simulink model "IEEE_39bus_genout"  (R2021a)
settings: Solver=ode3  StartTime=0.0  StopTime=100  FixedStep=Ts  MaxStep=1/60  RelTol=1e-2  AbsTol=1e-1
PreLoadFcn:
  | Ts=50e-6; ssn_ieee39_params; dec=20;
InitFcn:
  | Ts=50e-6; ssn_ieee39_params; dec=20;
values from neighbouring files (symbols this model uses):
  f = 50    [ssn_ieee39_params_ctrl.m]
  fNom = f    (= 60)    [ssn_ieee39_params_ctrl.m]
  ILR = 5.02    [ssn_ieee39_params_ctrl.m]
  IQMIN = 0.1    [ssn_ieee39_params_ctrl.m]
  ISCLIM = 1    [ssn_ieee39_params_ctrl.m]
  ITFpu = 1.10    (= 1.1)    [ssn_ieee39_params_ctrl.m]
  K = 1    [ssn_ieee39_params_ctrl.m]
  K1 = 1    [ssn_ieee39_params_ctrl.m]
  K2 = 2    [ssn_ieee39_params_ctrl.m]
  KCL = 1.04    [ssn_ieee39_params_ctrl.m]
  KFB = 0    [ssn_ieee39_params_ctrl.m]
  KFF = 1    [ssn_ieee39_params_ctrl.m]
  KFIX = 1    [ssn_ieee39_params_ctrl.m]
  KG = 1    [ssn_ieee39_params_ctrl.m]
  KIA = 59.91    [ssn_ieee39_params_ctrl.m]
  KIOEX = 0.0303    [ssn_ieee39_params_ctrl.m]
  KIUEX = 0.0303    [ssn_ieee39_params_ctrl.m]
  KIUOEX = 1    [ssn_ieee39_params_ctrl.m]
  KIUUEX = 1    [ssn_ieee39_params_ctrl.m]
  KLR = 22.47    [ssn_ieee39_params_ctrl.m]
  KM = 1    [ssn_ieee39_params_ctrl.m]
  KOEL = 0.24    [ssn_ieee39_params_ctrl.m]
  Kp = 1    [ssn_ieee39_params_ctrl.m]
  KPA = 30    [ssn_ieee39_params_ctrl.m]
  KPOEL = 1    [ssn_ieee39_params_ctrl.m]
  KPOEX = 0    [ssn_ieee39_params_ctrl.m]
  KPUEX = 0    [ssn_ieee39_params_ctrl.m]
  KSCALE = 0.319    [ssn_ieee39_params_ctrl.m]
  KUF = 0    [ssn_ieee39_params_ctrl.m]
  KUI = 0.001    [ssn_ieee39_params_ctrl.m]
  KUL = 0.24    [ssn_ieee39_params_ctrl.m]
  s = 10    [ssn_ieee39_params_ctrl.m]
  TA = 0.01    [ssn_ieee39_params_ctrl.m]
  Tadj = 0    [ssn_ieee39_params_ctrl.m]
  taps = [1 1 1.07 1.07 1.009 1.025 1 1.025 1.025 1.025]*1    [ssn_ieee39_params_ctrl.m]
  TF = 0.02    [ssn_ieee39_params_ctrl.m]
  TG = 0.024    [ssn_ieee39_params_ctrl.m]
  TINV = 0    [ssn_ieee39_params_ctrl.m]
  TIT = 0.1    [ssn_ieee39_params_ctrl.m]
  TL_10_11_len = 14    [ssn_ieee39_params_ctrl.m]
  TL_10_13_len = 14    [ssn_ieee39_params_ctrl.m]
  TL_13_14_len = 32    [ssn_ieee39_params_ctrl.m]
  TL_14_15_len = 70    [ssn_ieee39_params_ctrl.m]
  TL_15_16_len = 31.5    [ssn_ieee39_params_ctrl.m]
  TL_16_17_len = 26    [ssn_ieee39_params_ctrl.m]
  TL_16_19_len = 61    [ssn_ieee39_params_ctrl.m]
  TL_16_21_len = 46    [ssn_ieee39_params_ctrl.m]
  TL_16_24_len = 15    [ssn_ieee39_params_ctrl.m]
  TL_17_18_len = 26    [ssn_ieee39_params_ctrl.m]
  TL_17_27_len = 59    [ssn_ieee39_params_ctrl.m]
  TL_1_2_len = 134    [ssn_ieee39_params_ctrl.m]
  TL_1_39_len = 105    [ssn_ieee39_params_ctrl.m]
  TL_21_22_len = 47    [ssn_ieee39_params_ctrl.m]
  TL_22_23_len = 33    [ssn_ieee39_params_ctrl.m]
  TL_24_23_len = 88    [ssn_ieee39_params_ctrl.m]
  TL_25_26_len = 101    [ssn_ieee39_params_ctrl.m]
  TL_26_27_len = 46.5    [ssn_ieee39_params_ctrl.m]
  TL_26_28_len = 151    [ssn_ieee39_params_ctrl.m]
  TL_26_29_len = 200    [ssn_ieee39_params_ctrl.m]
  TL_28_29_len = 48    [ssn_ieee39_params_ctrl.m]
  TL_2_25_len = 28    [ssn_ieee39_params_ctrl.m]
  TL_2_2_len = 49    [ssn_ieee39_params_ctrl.m]
  TL_3_18_len = 42    [ssn_ieee39_params_ctrl.m]
  TL_3_4_len = 53    [ssn_ieee39_params_ctrl.m]
  TL_4_14_len = 33    [ssn_ieee39_params_ctrl.m]
  TL_4_5_len = 32.5    [ssn_ieee39_params_ctrl.m]
  TL_5_6_len = 14    [ssn_ieee39_params_ctrl.m]
  TL_5_8_len = 32    [ssn_ieee39_params_ctrl.m]
  TL_6_11_len = 26.5    [ssn_ieee39_params_ctrl.m]
  TL_6_7_len = 25.5    [ssn_ieee39_params_ctrl.m]
  TL_7_8_len = 15    [ssn_ieee39_params_ctrl.m]
  TL_8_9_len = 93    [ssn_ieee39_params_ctrl.m]
  TL_9_39_len = 136    [ssn_ieee39_params_ctrl.m]
  TOEL = 5.00    (= 5)    [ssn_ieee39_params_ctrl.m]
  TQREF = 0    [ssn_ieee39_params_ctrl.m]
  TQSCL = 0.012    [ssn_ieee39_params_ctrl.m]
  Ts_PMU = 1/1000    (= 0.001)    [ssn_ieee39_params_ctrl.m]
  TU1 = 0    [ssn_ieee39_params_ctrl.m]
  TU2 = 0    [ssn_ieee39_params_ctrl.m]
  TU3 = 0    [ssn_ieee39_params_ctrl.m]
  TU4 = 0    [ssn_ieee39_params_ctrl.m]
  TUL = 0    [ssn_ieee39_params_ctrl.m]
  TUP = 0.050    (= 0.05)    [ssn_ieee39_params_ctrl.m]
  TUQ = .005    (= 0.005)    [ssn_ieee39_params_ctrl.m]
  TUV = 0.2    [ssn_ieee39_params_ctrl.m]
  VAAMAX = VAMAX    (= 7.05)    [ssn_ieee39_params_ctrl.m]
  VAMAX = 7.05    [ssn_ieee39_params_ctrl.m]
  VAMIN = -6.11    [ssn_ieee39_params_ctrl.m]
  VBMAX = 999    [ssn_ieee39_params_ctrl.m]
  VF = 0    [ssn_ieee39_params_ctrl.m]
  VFB = 0    [ssn_ieee39_params_ctrl.m]
  VMMAX = 7.05    [ssn_ieee39_params_ctrl.m]
  VMMIN = -6.11    [ssn_ieee39_params_ctrl.m]
  VOELmax1 = 0.2353    [ssn_ieee39_params_ctrl.m]
  VOELmax2 = 0.0    (= 0)    [ssn_ieee39_params_ctrl.m]
  VOELmin1 = -0.24    [ssn_ieee39_params_ctrl.m]
  VOELmin2 = -1.0    (= -1)    [ssn_ieee39_params_ctrl.m]
  VRMAX = 7.05    [ssn_ieee39_params_ctrl.m]
  VRMIN = -6.11    [ssn_ieee39_params_ctrl.m]
  VSCLmax = 0.20    (= 0.2)    [ssn_ieee39_params_ctrl.m]
  VSCLmin = -0.10    (= -0.1)    [ssn_ieee39_params_ctrl.m]
  VUELmax1 = 1    [ssn_ieee39_params_ctrl.m]
  VUELmax2 = 1    [ssn_ieee39_params_ctrl.m]
  VUELmin1 = -1    [ssn_ieee39_params_ctrl.m]
  VUELmin2 = -1    [ssn_ieee39_params_ctrl.m]
  VUImax = 1    [ssn_ieee39_params_ctrl.m]
  VUImin = -1    [ssn_ieee39_params_ctrl.m]
undefined symbols (not defined in the file or in its folder): D1, Delta, MOV_segment9, powergui
libraries: spsThreePhaseVIMeasurementLib x42, slpidlib x40, powerlib_extras x30, op_dpl_lib x30, simulink_extras x20, spsST2AModel x20, spsThreePhaseParallelRLCLoadLib x19, spsThreePhaseTransformerTwoWindingsLib x13, spsSynchronousMachinepuStandardLib x10, simulink x10, spsPower3phInstantaneousLib x10, spsThreePhasePISectionLineLib x7
(part 6 of 12)

== system IEEE_39bus_genout/powergui/EquivalentModel4/Yout ==
  v,i : Inport
  Demux : Demux  Outputs=[2 1 1 1 1 1 1 1 1 1 1 1 1 1 1 1 1 1 1]
  tag scope: T61_5349_5543534420475=global, T61_5350_5545816817448=global, T61_5351_5548253508191=global, T61_5378_5534547660656=global, T61_5379_5536455134372=global, T61_5380_5538914352885=global, T62_5427_5653550607702=global, T62_5428_5655608975241=global, T62_5429_5658223434786=global, T73_6528_8854035683177=global, T83_7198_10636597834129=global, T83_7199_10636984207108=global, T83_7200_10631654038889=global, T83_7200_10637604369245=global, T83_7201_10632036892151=global, T83_7202_10632653534569=global, T84_7253_10872805404045=global, T84_7254_10873268569375=global, T84_7255_10873968878514=global
  wires:
  v,i/1 -> Demux/1
  Demux/1 -> [T73_6528_8854035683177]
  Demux/2 -> [T61_5378_5534547660656]
  Demux/3 -> [T61_5380_5538914352885]
  Demux/4 -> [T61_5379_5536455134372]
  Demux/5 -> [T62_5427_5653550607702]
  Demux/6 -> [T62_5429_5658223434786]
  Demux/7 -> [T62_5428_5655608975241]
  Demux/8 -> [T83_7198_10636597834129]
  Demux/9 -> [T83_7199_10636984207108]
  Demux/10 -> [T83_7200_10637604369245]
  Demux/11 -> [T84_7253_10872805404045]
  Demux/12 -> [T84_7254_10873268569375]
  Demux/13 -> [T84_7255_10873968878514]
  Demux/14 -> [T83_7200_10631654038889]
  Demux/15 -> [T83_7201_10632036892151]
  Demux/16 -> [T83_7202_10632653534569]
  Demux/17 -> [T61_5349_5543534420475]
  Demux/18 -> [T61_5350_5545816817448]
  Demux/19 -> [T61_5351_5548253508191]

== system IEEE_39bus_genout/powergui/EquivalentModel5/Sources ==
  Mux : Mux  Inputs=[1 1 1 1 1 1 1 1 1]
  u : Outport  VectorParamsAs1DForOutWhenUnconnected=off
  wires:
  Mux/1 -> u/1
  [T82_6942_9370736474068] -> Mux/1
  [T82_6943_9371870963565] -> Mux/2
  [T82_6944_9373248380867] -> Mux/3
  [T82_6945_9366351637990] -> Mux/4
  [T82_6946_9367479825753] -> Mux/5
  [T82_6947_9368850941320] -> Mux/6
  [T81_6895_9154721531022] -> Mux/7
  [T81_6896_9155759447410] -> Mux/8
  [T81_6897_9157036925528] -> Mux/9

== system IEEE_39bus_genout/powergui/EquivalentModel5/Yout ==
  v,i : Inport
  Demux : Demux  Outputs=[1 1 1 1 1 1 1 1 1 1 1 1]
  tag scope: T62_5429_5650937724339=global, T62_5430_5652992041777=global, T62_5431_5655602216520=global, T84_7253_10872378862689=global, T84_7254_10872842362976=global, T84_7255_10873543007073=global, T85_7300_11128438027275=global, T85_7301_11128992896359=global, T85_7302_11129788264501=global, T85_7303_11122740902331=global, T85_7304_11123289832852=global, T85_7305_11124079262431=global
  wires:
  v,i/1 -> Demux/1
  Demux/1 -> [T62_5429_5650937724339]
  Demux/2 -> [T62_5431_5655602216520]
  Demux/3 -> [T62_5430_5652992041777]
  Demux/4 -> [T85_7300_11128438027275]
  Demux/5 -> [T85_7301_11128992896359]
  Demux/6 -> [T85_7302_11129788264501]
  Demux/7 -> [T85_7303_11122740902331]
  Demux/8 -> [T85_7304_11123289832852]
  Demux/9 -> [T85_7305_11124079262431]
  Demux/10 -> [T84_7253_10872378862689]
  Demux/11 -> [T84_7254_10872842362976]
  Demux/12 -> [T84_7255_10873543007073]

== system IEEE_39bus_genout/powergui/EquivalentModel6/Sources ==
  Mux : Mux  Inputs=[1 1 1 1 1 1]
  u : Outport  VectorParamsAs1DForOutWhenUnconnected=off
  wires:
  Mux/1 -> u/1
  [T80_6854_8930207033252] -> Mux/1
  [T80_6855_8931137197264] -> Mux/2
  [T80_6856_8932303557277] -> Mux/3
  [T81_6907_9133741612475] -> Mux/4
  [T81_6908_9134756992429] -> Mux/5
  [T81_6909_9136011934111] -> Mux/6

== system IEEE_39bus_genout/powergui/EquivalentModel6/Yout ==
  v,i : Inport
  Demux : Demux  Outputs=[1 1 1 1 1 1 1 1 1]
  tag scope: T61_5385_5526707942377=global, T61_5386_5528601707568=global, T61_5387_5531046407508=global, T83_7212_10605693746042=global, T83_7213_10606055480996=global, T83_7214_10606651005107=global, T84_7265_10846924366936=global, T84_7266_10847366644693=global, T84_7267_10848046066259=global
  wires:
  v,i/1 -> Demux/1
  Demux/1 -> [T61_5385_5526707942377]
  Demux/2 -> [T61_5387_5531046407508]
  Demux/3 -> [T61_5386_5528601707568]
  Demux/4 -> [T83_7212_10605693746042]
  Demux/5 -> [T83_7213_10606055480996]
  Demux/6 -> [T83_7214_10606651005107]
  Demux/7 -> [T84_7265_10846924366936]
  Demux/8 -> [T84_7266_10847366644693]
  Demux/9 -> [T84_7267_10848046066259]

== system IEEE_39bus_genout/powergui/EquivalentModel7/Sources ==
  Mux : Mux  Inputs=[2 1 1 1 1 1 1]
  u : Outport  VectorParamsAs1DForOutWhenUnconnected=off
  wires:
  Mux/1 -> u/1
  [T71_6441_8457010710495] -> Mux/1
  [T82_6943_9370088412960] -> Mux/2
  [T82_6944_9371220372147] -> Mux/3
  [T82_6945_9372595259139] -> Mux/4
  [T81_6894_9156493190586] -> Mux/5
  [T81_6895_9157533469151] -> Mux/6
  [T81_6896_9158813309444] -> Mux/7

== system IEEE_39bus_genout/powergui/EquivalentModel7/Yout ==
  v,i : Inport
  Demux : Demux  Outputs=[2 1 1 1 1 1 1 1 1 1 1 1 1 1 1 1 1 1 1 1 1 1 1 1 1]
  tag scope: T61_5351_5540676149044=global, T61_5352_5542954377536=global, T61_5353_5545386899798=global, T62_5425_5656490020902=global, T62_5426_5654952364825=global, T62_5426_5658552253474=global, T62_5427_5653514430040=global, T62_5427_5657012618614=global, T62_5427_5661170802031=global, T62_5428_5652176216544=global, T62_5428_5655572705045=global, T62_5428_5659629073718=global, T62_5429_5650568630632=global, T62_5429_5654232512766=global, T62_5429_5658187066695=global, T62_5430_5652623040603=global, T62_5430_5656844780962=global, T62_5431_5655233313242=global, T71_6436_8387939612998=global, T84_7252_10874635314045=global, T84_7253_10875101038789=global, T84_7254_10875803907344=global, T85_7301_11127223259487=global, T85_7302_11127775744084=global, T85_7303_11128568727739=global
  wires:
  v,i/1 -> Demux/1
  Demux/1 -> [T71_6436_8387939612998]
  Demux/2 -> [T62_5425_5656490020902]
  Demux/3 -> [T62_5427_5661170802031]
  Demux/4 -> [T62_5426_5658552253474]
  Demux/5 -> [T62_5426_5654952364825]
  Demux/6 -> [T62_5428_5659629073718]
  Demux/7 -> [T62_5427_5657012618614]
  Demux/8 -> [T62_5427_5653514430040]
  Demux/9 -> [T62_5429_5658187066695]
  Demux/10 -> [T62_5428_5655572705045]
  Demux/11 -> [T62_5428_5652176216544]
  Demux/12 -> [T62_5430_5656844780962]
  Demux/13 -> [T62_5429_5654232512766]
  Demux/14 -> [T62_5429_5650568630632]
  Demux/15 -> [T62_5431_5655233313242]
  Demux/16 -> [T62_5430_5652623040603]
  Demux/17 -> [T85_7301_11127223259487]
  Demux/18 -> [T85_7302_11127775744084]
  Demux/19 -> [T85_7303_11128568727739]
  Demux/20 -> [T84_7252_10874635314045]
  Demux/21 -> [T84_7253_10875101038789]
  Demux/22 -> [T84_7254_10875803907344]
  Demux/23 -> [T61_5351_5540676149044]
  Demux/24 -> [T61_5352_5542954377536]
  Demux/25 -> [T61_5353_5545386899798]

== system IEEE_39bus_genout/powergui/EquivalentModel8/Sources ==
  Mux : Mux  Inputs=[1 1 1 1 1 1]
  u : Outport  VectorParamsAs1DForOutWhenUnconnected=off
  wires:
  Mux/1 -> u/1
  [T82_6944_9367002881001] -> Mux/1
  [T82_6945_9368133599074] -> Mux/2
  [T82_6946_9369507244952] -> Mux/3
  [T82_6947_9362805089533] -> Mux/4
  [T82_6948_9363929505872] -> Mux/5
  [T82_6949_9365296850015] -> Mux/6

== system IEEE_39bus_genout/powergui/EquivalentModel8/Yout ==
  v,i : Inport
  Demux : Demux  Outputs=[1 1 1 1 1 1 1 1 1]
  tag scope: T62_5430_5649798953424=global, T62_5431_5651851292078=global, T62_5432_5654459373369=global, T85_7302_11123958630090=global, T85_7303_11124509945098=global, T85_7304_11125301759165=global, T85_7305_11118442139291=global, T85_7306_11118987515737=global, T85_7307_11119773391241=global
  wires:
  v,i/1 -> Demux/1
  Demux/1 -> [T62_5430_5649798953424]
  Demux/2 -> [T62_5432_5654459373369]
  Demux/3 -> [T62_5431_5651851292078]
  Demux/4 -> [T85_7302_11123958630090]
  Demux/5 -> [T85_7303_11124509945098]
  Demux/6 -> [T85_7304_11125301759165]
  Demux/7 -> [T85_7305_11118442139291]
  Demux/8 -> [T85_7306_11118987515737]
  Demux/9 -> [T85_7307_11119773391241]

== system IEEE_39bus_genout/powergui/EquivalentModel9/Sources ==
  Mux : Mux  Inputs=[1 1 1 1 1 1 1 1 1 1 1 1 1 1 1]
  u : Outport  VectorParamsAs1DForOutWhenUnconnected=off
  wires:
  Mux/1 -> u/1
  [T82_6946_9363459514447] -> Mux/1
  [T82_6947_9364586461096] -> Mux/2
  [T82_6948_9365956335550] -> Mux/3
  [T82_6948_9360106374407] -> Mux/4
  [T82_6949_9361229549631] -> Mux/5
  [T82_6950_9362595652660] -> Mux/6
  [T82_6950_9357536452456] -> Mux/7
  [T82_6951_9358655660923] -> Mux/8
  [T82_6952_9360017797195] -> Mux/9
  [T82_6943_9368326571406] -> Mux/10
  [T82_6944_9369459702590] -> Mux/11
  [T82_6945_9370835761578] -> Mux/12
  [T82_6946_9362714806637] -> Mux/13
  [T82_6947_9363841987684] -> Mux/14
  [T82_6948_9365212096537] -> Mux/15

== system IEEE_39bus_genout/powergui/EquivalentModel9/Yout ==
  v,i : Inport
  Demux : Demux  Outputs=[1 1 1 1 1 1 1 1 1 1 1 1 1 1 1 1 1 1]
  tag scope: T62_5431_5648759903800=global, T62_5432_5650810263670=global, T62_5433_5653416251507=global, T85_7301_11125797541042=global, T85_7302_11126351130092=global, T85_7303_11127145218202=global, T85_7304_11118999341378=global, T85_7304_11119662827022=global, T85_7305_11119547323202=global, T85_7305_11120210587955=global, T85_7306_11115550618073=global, T85_7306_11120335804084=global, T85_7306_11120998847947=global, T85_7307_11116094824930=global, T85_7308_11112148312527=global, T85_7308_11116879530846=global, T85_7309_11112688781232=global, T85_7310_11113469748997=global
  wires:
  v,i/1 -> Demux/1
  Demux/1 -> [T62_5431_5648759903800]
  Demux/2 -> [T62_5433_5653416251507]
  Demux/3 -> [T62_5432_5650810263670]
  Demux/4 -> [T85_7304_11119662827022]
  Demux/5 -> [T85_7305_11120210587955]
  Demux/6 -> [T85_7306_11120998847947]
  Demux/7 -> [T85_7306_11115550618073]
  Demux/8 -> [T85_7307_11116094824930]
  Demux/9 -> [T85_7308_11116879530846]
  Demux/10 -> [T85_7308_11112148312527]
  Demux/11 -> [T85_7309_11112688781232]
  Demux/12 -> [T85_7310_11113469748997]
  Demux/13 -> [T85_7301_11125797541042]
  Demux/14 -> [T85_7302_11126351130092]
  Demux/15 -> [T85_7303_11127145218202]
  Demux/16 -> [T85_7304_11118999341378]
  Demux/17 -> [T85_7305_11119547323202]
  Demux/18 -> [T85_7306_11120335804084]

== system IEEE_39bus_genout/SM_master/G1/G1/Generator Measurements (Output) ==
  note: (It2nd)
  note: (QT2nd)
  note: (PT2nd)
  note: Stator Current
  note: Reactive Power
  note: Active Power
  note: Note:
      | This block splits the combined measurement signal into the individual parameter signals.
  note: Selected
      | Synchronous Machine
      | Measurement Outputs
      | (Recombined)
  note: Stator Voltage
  note: Rotor Speed
  note: Field Current
  m : Inport
  Bus Creator : BusCreator  Inputs=7
  Bus Selector : BusSelector  OutputSignals="Mechanical.Electrical power  Pe (pu),Mechanical.Rotor speed  wm  (pu),Output active power   Peo (pu),Output reactive power  Qeo (pu),dq0 components.Stator current  id (pu),dq0 components.Stator current  iq (pu)"
  Bus Selector1 : BusSelector  OutputSignals="dq0 components.Stator voltage  vq (pu),dq0 components.Stator voltage  vd (pu)"
  Bus Selector2 : BusSelector  OutputSignals="Mechanical.Rotor speed  wm  (pu),dq0 components.Field current  ifd (pu)"
  Fcn1 : Fcn  Expr=sqrt(u(1)^2 + u(2)^2)
  Hypot : Math  Operator=hypot  SaturateOnIntegerOverflow=on
  Mux : Mux  Inputs=2
  to W : Gain  Gain=Pn
  to W1 : Gain  Gain=Pn
  to W2 : Gain  Gain=Pn
  sm : Outport  VectorParamsAs1DForOutWhenUnconnected=off
  wm : Outport  Port=2  VectorParamsAs1DForOutWhenUnconnected=off
  Vt : Outport  Port=3  VectorParamsAs1DForOutWhenUnconnected=off
  Ifd : Outport  Port=4  VectorParamsAs1DForOutWhenUnconnected=off
  It : Outport  Port=5  VectorParamsAs1DForOutWhenUnconnected=off
  PT : Outport  Port=6  VectorParamsAs1DForOutWhenUnconnected=off
  QT : Outport  Port=7  VectorParamsAs1DForOutWhenUnconnected=off
  wires:
  Bus Selector/4 -> to W2/1, QT/1, Bus Creator/5  "<Output reactive power  Qeo (pu)>"
  Bus Selector/1 -> Bus Creator/2, to W/1  "<Electrical power  Pe (pu)>"
  Bus Selector/3 -> to W1/1, PT/1, Bus Creator/4  "<Output active power   Peo (pu)>"
  to W/1 -> Bus Creator/1  "Electrical Power (W)"
  Bus Creator/1 -> sm/1
  Bus Selector/2 -> Bus Creator/3  "<Rotor speed  wm  (pu)>"
  to W1/1 -> Bus Creator/6  "Active Power (W)"
  to W2/1 -> Bus Creator/7  "Reactive Power (W)"
  Bus Selector/5 -> Hypot/1  "<Stator current  id (pu)>"
  Bus Selector/6 -> Hypot/2  "<Stator current  iq (pu)>"
  Hypot/1 -> It/1
  Bus Selector2/2 -> Ifd/1  "<Field current  ifd (pu)>"
  Bus Selector2/1 -> wm/1  "<Rotor speed  wm  (pu)>"
  m/1 -> Bus Selector/1, Bus Selector1/1, Bus Selector2/1
  Fcn1/1 -> Vt/1  "Stator Voltage (pu)"
  Bus Selector1/1 -> Mux/1  "<Stator voltage  vq (pu)>"
  Bus Selector1/2 -> Mux/2  "<Stator voltage  vd (pu)>"
  Mux/1 -> Fcn1/1

== system IEEE_39bus_genout/SM_master/G1/G1/Governor model with Droop ==
  note: Tg = Governor time constant
  wref (pu)1 : Inport
  w (pu) : Inport  Port=2
  Input : Inport  Port=3
  1/(1+sTg) : TransferFcn  Denominator=[0.02 1]
  1/R : Gain  Gain=1/0.05
  Scope{2..6,8} (6 alike) : Scope
  Sum : Sum  Inputs=|-+
  Sum1 : Sum  Inputs=|-+
  Pmec (pu) : Outport  InitialOutput=0  VectorParamsAs1DForOutWhenUnconnected=off
  wires:
  w (pu)/1 -> Scope8/1, Sum/2
  1/R/1 -> Scope4/1, Sum1/1
  Sum1/1 -> Scope2/1, 1/(1+sTg)/1
  Sum/1 -> Scope3/1, 1/R/1
  wref (pu)1/1 -> Sum/1
  1/(1+sTg)/1 -> Scope5/1, Pmec (pu)/1
  Input/1 -> Sum1/2, Scope6/1

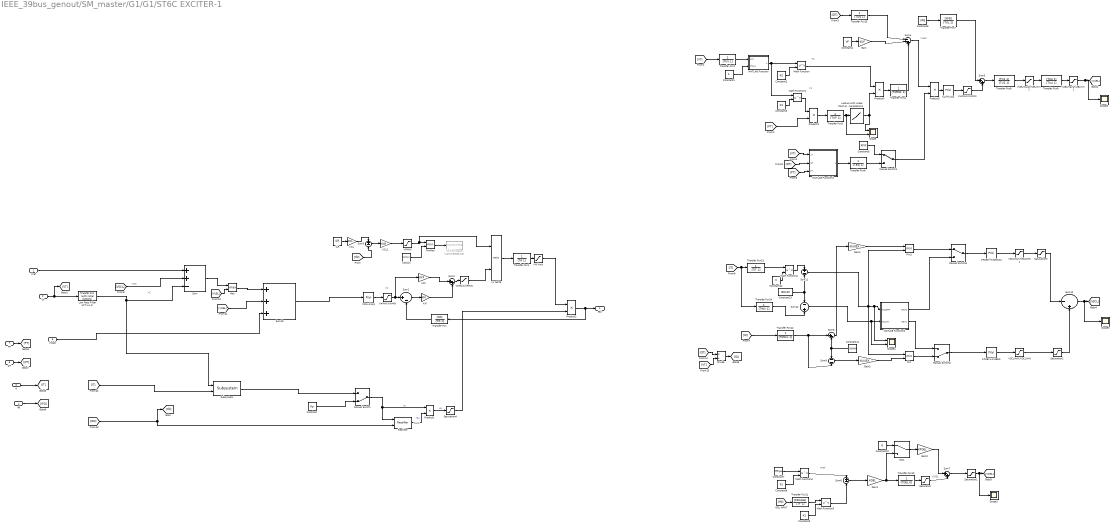
== system IEEE_39bus_genout/SM_master/G1/G1/ST6C EXCITER-1 ==
  note: VC
  note: VIOEL
  note: IFref
  note: VUerr
  note: F1
  note: F2
  note: VA
  note: Fex0
  note: VR0
  Vref : Inport
  Vt : Inport  Port=2
  It : Inport  Port=3
  Ifd : Inport  Port=4
  Vstab : Inport  Port=5
  QT : Inport  Port=6
  PT : Inport  Port=7
  Constant : Constant  Value=Kp
  Constant1 : Constant
  Constant10 : Constant  Value=0
  Constant11 : Constant  Value=IQMIN
  Constant12 : Constant  Value=K
  Constant13 : Constant  Value=ISCLIM
  Constant2 : Constant  Value=K2
  Constant3 : Constant  Value=K1
  Constant4 : Constant  Value=VF
  Constant5 : Constant  Value=KFIX
  Constant6 : Constant  Value=VFB
  Constant7 : Constant  Value=ITFpu
  Constant8 : Constant  Value=K1
  Constant9 : Constant  Value=K1
  Divide : Product  Inputs=*/
  Gain : Gain  Gain=KUF
  Gain1 : Gain  Gain=KOEL
  Gain2 : Gain  Gain=KPOEL
  Gain3 : Gain  Gain=KIUUEX
  Gain4 : Gain  Gain=KIUOEX
  ILR : Constant  Value=ILR
  KCL : Gain  Gain=KCL
  KCL1 : Gain  Gain=KLR
  KFF : Gain  Gain=KFF
  KM : Gain  Gain=KM
  KPA+KIA/s : slpidlib/PID Controller  Controller=PI  Form=Parallel  TimeDomain=Continuous-time  UseExternalTs=off  SampleTime=-1  IntegratorMethod=Forward Euler  FilterMethod=Forward Euler  ControllerParametersSource=internal  P=KPA  I=KIA  D=0  UseFilter=on  N=100  TunerSelectOption=Transfer Function Based (PID Tuner App)  InitialConditionSource=internal  InitialConditionForIntegrator=0  InitialConditionForFilter=0  DifferentiatorICPrevScaledInput=0  ExternalReset=none  TrackingMode=off  Kt=1  LimitOutput=off  SatLimitsSource=internal  UpperSaturationLimit=inf  LowerSaturationLimit=-inf  LinearizeAsGain=on  AntiWindupMode=none  Kb=1  POutMin=[]  POutMax=[]  IOutMin=[]  IOutMax=[]  DOutMin=[]  DOutMax=[]  NOutMin=[]  NOutMax=[]  SumOutMin=[]  SumOutMax=[]  SaturationOutMin=[]  SaturationOutMax=[]  PParamMin=[]  PParamMax=[]  IParamMin=[]  IParamMax=[]  DParamMin=[]  DParamMax=[]  NParamMin=[]  NParamMax=[]  KbParamMin=[]  KbParamMax=[]  KtParamMin=[]  KtParamMax=[]  KbOutMin=[]  KbOutMax=[]  KtOutMin=[]  KtOutMax=[]  IntegratorOutMin=[]  IntegratorOutMax=[]  FilterOutMin=[]  FilterOutMax=[]  SumI1OutMin=[]  SumI1OutMax=[]  SumI2OutMin=[]  SumI2OutMax=[]  SumI3OutMin=[]  SumI3OutMax=[]  SumI4OutMin=[]  SumI4OutMax=[]  SumDOutMin=[]  SumDOutMax=[]  DifferentiatorOutMin=[]  DifferentiatorOutMax=[]  FilterDiffOutCoefMin=[]  FilterDiffOutCoefMax=[]  ReciprocalOutMin=[]  ReciprocalOutMax=[]  SumDenOutMin=[]  SumDenOutMax=[]  SumNumOutMin=[]  SumNumOutMax=[]  DivideOutMin=[]  DivideOutMax=[]  UdiffTsProdOutMin=[]  UdiffTsProdOutMax=[]  NTsProdOutMin=[]  NTsProdOutMax=[]  UintegralTsProdOutMin=[]  UintegralTsProdOutMax=[]  UngainTsProdOutMin=[]  UngainTsProdOutMax=[]  IntegratorContinuousStateAttributes=''  IntegratorStateMustResolveToSignalObject=off  IntegratorRTWStateStorageClass=Auto  FilterContinuousStateAttributes=''  FilterStateMustResolveToSignalObject=off  FilterRTWStateStorageClass=Auto  ParallelPVariant=InternalParameters  IdealPVariant=Disabled  IVariant=InternalParameters  DVariant=Disabled  IntegratorVariant=Continuous  SatVariant=Disabled  AWVariant=Passthrough  PCopyVariant=Disabled  TRVariant=Disabled  FdbkBlocksVariant=Forward  IdealPFdbkVariant=Disabled  SatFdbkVariant=Disabled  DerivativeFilterVariant=Disabled  NVariant=Disabled  NCopyVariant=Disabled_SignalSpec  FilterICVariant=Disabled  IntegratorICVariant=InternalICs  ExternalResetVariant=Disabled  TRSumVariant=Passthrough  SumFdbkVariant=Disabled  SumVariant=Sum_PI  TsampFilterVariant=InternalTs  TsampNgainVariant=Passthrough  TsampIntegralVariant=Passthrough  ExternalSaturationOutDataTypeStr=Inherit: Same as second input
  KPOEX+KIOEX/S1 : slpidlib/PID Controller  Controller=PI  Form=Parallel  TimeDomain=Continuous-time  UseExternalTs=off  SampleTime=-1  IntegratorMethod=Forward Euler  FilterMethod=Forward Euler  ControllerParametersSource=internal  P=KPOEX  I=KIOEX  D=0  UseFilter=on  N=100  TunerSelectOption=Transfer Function Based (PID Tuner App)  InitialConditionSource=internal  InitialConditionForIntegrator=0  InitialConditionForFilter=0  DifferentiatorICPrevScaledInput=0  ExternalReset=none  TrackingMode=off  Kt=1  LimitOutput=off  SatLimitsSource=internal  UpperSaturationLimit=inf  LowerSaturationLimit=-inf  LinearizeAsGain=on  AntiWindupMode=none  Kb=1  POutMin=[]  POutMax=[]  IOutMin=[]  IOutMax=[]  DOutMin=[]  DOutMax=[]  NOutMin=[]  NOutMax=[]  SumOutMin=[]  SumOutMax=[]  SaturationOutMin=[]  SaturationOutMax=[]  PParamMin=[]  PParamMax=[]  IParamMin=[]  IParamMax=[]  DParamMin=[]  DParamMax=[]  NParamMin=[]  NParamMax=[]  KbParamMin=[]  KbParamMax=[]  KtParamMin=[]  KtParamMax=[]  KbOutMin=[]  KbOutMax=[]  KtOutMin=[]  KtOutMax=[]  IntegratorOutMin=[]  IntegratorOutMax=[]  FilterOutMin=[]  FilterOutMax=[]  SumI1OutMin=[]  SumI1OutMax=[]  SumI2OutMin=[]  SumI2OutMax=[]  SumI3OutMin=[]  SumI3OutMax=[]  SumI4OutMin=[]  SumI4OutMax=[]  SumDOutMin=[]  SumDOutMax=[]  DifferentiatorOutMin=[]  DifferentiatorOutMax=[]  FilterDiffOutCoefMin=[]  FilterDiffOutCoefMax=[]  ReciprocalOutMin=[]  ReciprocalOutMax=[]  SumDenOutMin=[]  SumDenOutMax=[]  SumNumOutMin=[]  SumNumOutMax=[]  DivideOutMin=[]  DivideOutMax=[]  UdiffTsProdOutMin=[]  UdiffTsProdOutMax=[]  NTsProdOutMin=[]  NTsProdOutMax=[]  UintegralTsProdOutMin=[]  UintegralTsProdOutMax=[]  UngainTsProdOutMin=[]  UngainTsProdOutMax=[]  IntegratorContinuousStateAttributes=''  IntegratorStateMustResolveToSignalObject=off  IntegratorRTWStateStorageClass=Auto  FilterContinuousStateAttributes=''  FilterStateMustResolveToSignalObject=off  FilterRTWStateStorageClass=Auto  ParallelPVariant=InternalParameters  IdealPVariant=Disabled  IVariant=InternalParameters  DVariant=Disabled  IntegratorVariant=Continuous  SatVariant=Disabled  AWVariant=Passthrough  PCopyVariant=Disabled  TRVariant=Disabled  FdbkBlocksVariant=Forward  IdealPFdbkVariant=Disabled  SatFdbkVariant=Disabled  DerivativeFilterVariant=Disabled  NVariant=Disabled  NCopyVariant=Disabled_SignalSpec  FilterICVariant=Disabled  IntegratorICVariant=InternalICs  ExternalResetVariant=Disabled  TRSumVariant=Passthrough  SumFdbkVariant=Disabled  SumVariant=Sum_PI  TsampFilterVariant=InternalTs  TsampNgainVariant=Passthrough  TsampIntegralVariant=Passthrough  ExternalSaturationOutDataTypeStr=Inherit: Same as second input
  KPUEX+KIUES/S : slpidlib/PID Controller  Controller=PI  Form=Parallel  TimeDomain=Continuous-time  UseExternalTs=off  SampleTime=-1  IntegratorMethod=Forward Euler  FilterMethod=Forward Euler  ControllerParametersSource=internal  P=KPUEX  I=KIUEX  D=0  UseFilter=on  N=100  TunerSelectOption=Transfer Function Based (PID Tuner App)  InitialConditionSource=internal  InitialConditionForIntegrator=0  InitialConditionForFilter=0  DifferentiatorICPrevScaledInput=0  ExternalReset=none  TrackingMode=off  Kt=1  LimitOutput=off  SatLimitsSource=internal  UpperSaturationLimit=inf  LowerSaturationLimit=-inf  LinearizeAsGain=on  AntiWindupMode=none  Kb=1  POutMin=[]  POutMax=[]  IOutMin=[]  IOutMax=[]  DOutMin=[]  DOutMax=[]  NOutMin=[]  NOutMax=[]  SumOutMin=[]  SumOutMax=[]  SaturationOutMin=[]  SaturationOutMax=[]  PParamMin=[]  PParamMax=[]  IParamMin=[]  IParamMax=[]  DParamMin=[]  DParamMax=[]  NParamMin=[]  NParamMax=[]  KbParamMin=[]  KbParamMax=[]  KtParamMin=[]  KtParamMax=[]  KbOutMin=[]  KbOutMax=[]  KtOutMin=[]  KtOutMax=[]  IntegratorOutMin=[]  IntegratorOutMax=[]  FilterOutMin=[]  FilterOutMax=[]  SumI1OutMin=[]  SumI1OutMax=[]  SumI2OutMin=[]  SumI2OutMax=[]  SumI3OutMin=[]  SumI3OutMax=[]  SumI4OutMin=[]  SumI4OutMax=[]  SumDOutMin=[]  SumDOutMax=[]  DifferentiatorOutMin=[]  DifferentiatorOutMax=[]  FilterDiffOutCoefMin=[]  FilterDiffOutCoefMax=[]  ReciprocalOutMin=[]  ReciprocalOutMax=[]  SumDenOutMin=[]  SumDenOutMax=[]  SumNumOutMin=[]  SumNumOutMax=[]  DivideOutMin=[]  DivideOutMax=[]  UdiffTsProdOutMin=[]  UdiffTsProdOutMax=[]  NTsProdOutMin=[]  NTsProdOutMax=[]  UintegralTsProdOutMin=[]  UintegralTsProdOutMax=[]  UngainTsProdOutMin=[]  UngainTsProdOutMax=[]  IntegratorContinuousStateAttributes=''  IntegratorStateMustResolveToSignalObject=off  IntegratorRTWStateStorageClass=Auto  FilterContinuousStateAttributes=''  FilterStateMustResolveToSignalObject=off  FilterRTWStateStorageClass=Auto  ParallelPVariant=InternalParameters  IdealPVariant=Disabled  IVariant=InternalParameters  DVariant=Disabled  IntegratorVariant=Continuous  SatVariant=Disabled  AWVariant=Passthrough  PCopyVariant=Disabled  TRVariant=Disabled  FdbkBlocksVariant=Forward  IdealPFdbkVariant=Disabled  SatFdbkVariant=Disabled  DerivativeFilterVariant=Disabled  NVariant=Disabled  NCopyVariant=Disabled_SignalSpec  FilterICVariant=Disabled  IntegratorICVariant=InternalICs  ExternalResetVariant=Disabled  TRSumVariant=Passthrough  SumFdbkVariant=Disabled  SumVariant=Sum_PI  TsampFilterVariant=InternalTs  TsampNgainVariant=Passthrough  TsampIntegralVariant=Passthrough  ExternalSaturationOutDataTypeStr=Inherit: Same as second input
  KUI+KUI/s : slpidlib/PID Controller  Controller=PI  Form=Parallel  TimeDomain=Continuous-time  UseExternalTs=off  SampleTime=-1  IntegratorMethod=Forward Euler  FilterMethod=Forward Euler  ControllerParametersSource=internal  P=KUL  I=KUI  D=0  UseFilter=on  N=100  TunerSelectOption=Transfer Function Based (PID Tuner App)  InitialConditionSource=internal  InitialConditionForIntegrator=0  InitialConditionForFilter=0  DifferentiatorICPrevScaledInput=0  ExternalReset=none  TrackingMode=off  Kt=1  LimitOutput=off  SatLimitsSource=internal  UpperSaturationLimit=inf  LowerSaturationLimit=-inf  LinearizeAsGain=on  AntiWindupMode=none  Kb=1  POutMin=[]  POutMax=[]  IOutMin=[]  IOutMax=[]  DOutMin=[]  DOutMax=[]  NOutMin=[]  NOutMax=[]  SumOutMin=[]  SumOutMax=[]  SaturationOutMin=[]  SaturationOutMax=[]  PParamMin=[]  PParamMax=[]  IParamMin=[]  IParamMax=[]  DParamMin=[]  DParamMax=[]  NParamMin=[]  NParamMax=[]  KbParamMin=[]  KbParamMax=[]  KtParamMin=[]  KtParamMax=[]  KbOutMin=[]  KbOutMax=[]  KtOutMin=[]  KtOutMax=[]  IntegratorOutMin=[]  IntegratorOutMax=[]  FilterOutMin=[]  FilterOutMax=[]  SumI1OutMin=[]  SumI1OutMax=[]  SumI2OutMin=[]  SumI2OutMax=[]  SumI3OutMin=[]  SumI3OutMax=[]  SumI4OutMin=[]  SumI4OutMax=[]  SumDOutMin=[]  SumDOutMax=[]  DifferentiatorOutMin=[]  DifferentiatorOutMax=[]  FilterDiffOutCoefMin=[]  FilterDiffOutCoefMax=[]  ReciprocalOutMin=[]  ReciprocalOutMax=[]  SumDenOutMin=[]  SumDenOutMax=[]  SumNumOutMin=[]  SumNumOutMax=[]  DivideOutMin=[]  DivideOutMax=[]  UdiffTsProdOutMin=[]  UdiffTsProdOutMax=[]  NTsProdOutMin=[]  NTsProdOutMax=[]  UintegralTsProdOutMin=[]  UintegralTsProdOutMax=[]  UngainTsProdOutMin=[]  UngainTsProdOutMax=[]  IntegratorContinuousStateAttributes=''  IntegratorStateMustResolveToSignalObject=off  IntegratorRTWStateStorageClass=Auto  FilterContinuousStateAttributes=''  FilterStateMustResolveToSignalObject=off  FilterRTWStateStorageClass=Auto  ParallelPVariant=InternalParameters  IdealPVariant=Disabled  IVariant=InternalParameters  DVariant=Disabled  IntegratorVariant=Continuous  SatVariant=Disabled  AWVariant=Passthrough  PCopyVariant=Disabled  TRVariant=Disabled  FdbkBlocksVariant=Forward  IdealPFdbkVariant=Disabled  SatFdbkVariant=Disabled  DerivativeFilterVariant=Disabled  NVariant=Disabled  NCopyVariant=Disabled_SignalSpec  FilterICVariant=Disabled  IntegratorICVariant=InternalICs  ExternalResetVariant=Disabled  TRSumVariant=Passthrough  SumFdbkVariant=Disabled  SumVariant=Sum_PI  TsampFilterVariant=InternalTs  TsampNgainVariant=Passthrough  TsampIntegralVariant=Passthrough  ExternalSaturationOutDataTypeStr=Inherit: Same as second input
  LV GATE : MinMax  Inputs=2
  Lookup with Linear Point-slope Interpolation1 : Lookup_n-D  NumberOfTableDimensions=1  BreakpointsForDimension1=[0 1]  BreakpointsForDimension2=[-0.29 0.58]  Table="[-0.29  0]"  InternalRulePriority=Speed  RndMeth=Simplest  InputSameDT=on
  Low Pass Filter 1/(Tr.s+1) : simulink_extras/Additional Linear/Transfer Fcn (with initial outputs)  N=1  D=[0.016 1]  Y0=Vt0  U0=Vt0
  MATLAB Function : MATLAB Function  TreatAsAtomicUnit=on
  MATLAB Function1 : MATLAB Function  TreatAsAtomicUnit=on
  MATLAB Function2 : MATLAB Function  TreatAsAtomicUnit=on
  Manual Switch : ManualSwitch  CurrentSetting=0
  Manual Switch1 : ManualSwitch
  Manual Switch2 : ManualSwitch  CurrentSetting=0
  Manual Switch3 : ManualSwitch
  Math Function{,1..4} (5 alike) : Math  Operator=pow  SignedPower=on  SaturateOnIntegerOverflow=on
  Max : MinMax  Function=max  Inputs=2
  Min : MinMax  Inputs=2
  Min1 : MinMax  Inputs=2
  MinMax : MinMax  Inputs=2
  Product{1..5} (5 alike) : Product  InputSameDT=on  RndMeth=Zero  SaturateOnIntegerOverflow=on  OutDataTypeStr=Inherit: Same as first input
  Rectifier : spsST2AModel/Continuous/Rectifier  Kc=Kc
      settings: SourceProductBaseCode=PS
  SW1 : ManualSwitch
  Saturation : Saturate  UpperLimit=VOELmax1  LowerLimit=VOELmin1
  Saturation1 : Saturate  UpperLimit=VOELmax2  LowerLimit=VOELmin2
  Saturation2 : Saturate  UpperLimit=inf  LowerLimit=0
  Saturation3 : Saturate  UpperLimit=inf  LowerLimit=0
  Saturation4 : Saturate  UpperLimit=VBMAX  LowerLimit=eps
  Scope : Scope  NumInputPorts=2
  Scope1 : Scope
  Scope2 : Scope
  Scope3 : Scope
  Scope4 : Scope  NumInputPorts=2
  Subsystem : spsST2AModel/Continuous/Subsystem  KI=KI  Kp=Kp
      settings: SourceProductBaseCode=PS
  Sum : Sum  Inputs=++-  InputSameDT=on  SaturateOnIntegerOverflow=on  OutDataTypeStr=Inherit: Same as first input
  Sum1 : Sum  Inputs=|+-
  Sum10 : Sum  Inputs=|-+
  Sum11 : Sum  Inputs=+-
  Sum12 : Sum  Inputs=-+
  Sum13 : Sum  Inputs=+++  InputSameDT=on  SaturateOnIntegerOverflow=on  OutDataTypeStr=Inherit: Same as first input
  Sum2 : Sum  Inputs=|++
  Sum3 : Sum  Inputs=+-
  Sum4 : Sum  Inputs=|--+
  Sum5 : Sum  Inputs=|++
  Sum6 : Sum  Inputs=+-
  Sum7 : Sum  Inputs=|++
  Sum8 : Sum  Inputs=|+-
  Sum9 : Sum  Inputs=--
  To Workspace : ToWorkspace  Commented=on  VariableName=VAAMAXSWa  SaveFormat=Timeseries  SampleTime=-1
  Transfer Fcn : TransferFcn  Numerator=[KG]  Denominator=[TG 1]
  Transfer Fcn1 : TransferFcn  Denominator=[TA 1]
  Transfer Fcn10 : TransferFcn  Denominator=[TOEL 0]
  Transfer Fcn11 : TransferFcn  Numerator=[KSCALE]  Denominator=[TF 1]
  Transfer Fcn12 : TransferFcn  Denominator=[TQSCL 1]
  Transfer Fcn13 : TransferFcn  Denominator=[TIT 1]
  Transfer Fcn14 : TransferFcn  Denominator=[TINV 1]
  Transfer Fcn15 : TransferFcn  Denominator=[TUQ 1]
  Transfer Fcn2 : TransferFcn  Denominator=[TUV 1]
  Transfer Fcn3 : TransferFcn  Denominator=[TUP 1]
  Transfer Fcn4 : TransferFcn  Denominator=[TQREF 1]
  Transfer Fcn6 : TransferFcn  Denominator=[Tadj 1]
  Transfer Fcn7 : TransferFcn  Numerator=[KFB]  Denominator=[TUL 1]
  Transfer Fcn8 : TransferFcn  Numerator=[TU1 1]  Denominator=[TU2 1]
  Transfer Fcn9 : TransferFcn  Numerator=[TU3 1]  Denominator=[TU4 1]
  "VAMAX " : Constant  Value=VAMAX
  VAMAX/VAMIN : Saturate  UpperLimit=VAAMAX  LowerLimit=VAMIN
  VM limit : Saturate  UpperLimit=VMMAX  LowerLimit=VMMIN
  VRMAX/VRMIN : Saturate  UpperLimit=VRMAX  LowerLimit=VRMIN
  VRMIN : Saturate  UpperLimit=inf  LowerLimit=VRMIN
  VSCLMAX/VSCLMIN : Saturate  UpperLimit=VSCLmax  LowerLimit=VSCLmin
  VSCLMAX/VSCLMIN1 : Saturate  UpperLimit=VSCLmax  LowerLimit=VSCLmin
  VUELmax1/VUELmin1 : Saturate  UpperLimit=VUELmax1  LowerLimit=VUELmin1
  "VUELmax2/VUELmin2 " : Saturate  UpperLimit=VUELmax2  LowerLimit=VUELmin2
  VUIMAX/VUIMIN : Saturate  UpperLimit=VUImax  LowerLimit=VUImin
  Efd : Outport  VectorParamsAs1DForOutWhenUnconnected=off
  wires:
  VM limit/1 -> Product2/1
  MinMax/1 -> To Workspace/1
  "VAMAX "/1 -> MinMax/2
  Transfer Fcn1/1 -> VM limit/1
  [VSCL] -> Sum/2
  KPA+KIA/s/1 -> VAMAX/VAMIN/1
  Subsystem/1 -> Manual Switch/1
  Manual Switch/1 -> Product1/1, Rectifier/1  "Ve"
  Product1/1 -> Saturation4/1  "VB"
  [IFD] -> [Ifd], Rectifier/2
  Rectifier/1 -> Product1/2  "Fex"
  Sum2/1 -> VRMAX/VRMIN/1
  Vt/1 -> [VT], Low Pass Filter 1/(Tr.s+1)/1
  Vstab/1 -> Sum13/3
  [IT] -> Subsystem/2
  Vref/1 -> Sum/1
  Constant/1 -> Manual Switch/2
  Transfer Fcn/1 -> Sum1/2
  Sum1/1 -> KM/1
  Low Pass Filter 1/(Tr.s+1)/1 -> Subsystem/1, Sum/3
  Product2/1 -> Efd/1, Transfer Fcn/1
  VRMAX/VRMIN/1 -> LV GATE/2
  Sum/1 -> Max/1
  KFF/1 -> Sum2/1
  KCL/1 -> Sum3/1
  KM/1 -> Sum2/2
  ILR/1 -> KCL/1
  Sum3/1 -> KCL1/1
  [Ifd] -> Sum3/2
  VRMIN/1 -> LV GATE/1, MinMax/1
  VAMAX/VAMIN/1 -> KFF/1, Sum1/1
  LV GATE/1 -> Transfer Fcn1/1
  [VT] -> Transfer Fcn2/1
  Transfer Fcn2/1 -> MATLAB Function/1(VTF)
  Constant1/1 -> MATLAB Function/2(Vbias)
  MATLAB Function/1(u) -> Math Function1/1, Math Function/1
  Constant2/1 -> Math Function/2
  Math Function/1 -> Product4/1
  Constant3/1 -> Math Function1/2
  Math Function1/1 -> Product3/1
  [PT] -> Product3/2
  Product3/1 -> Transfer Fcn3/1
  Transfer Fcn3/1 -> Scope/2, Lookup with Linear Point-slope Interpolation1/1
  Lookup with Linear Point-slope Interpolation1/1 -> Scope/1, Product4/2
  Product4/1 -> Transfer Fcn4/1
  KUI+KUI/s/1 -> VUIMAX/VUIMIN/1
  Transfer Fcn4/1 -> Sum4/3
  Constant4/1 -> Gain/1
  Gain/1 -> Sum4/2
  [QT] -> Transfer Fcn15/1
  Transfer Fcn15/1 -> Sum4/1
  Sum4/1 -> Product5/1
  Product5/1 -> KUI+KUI/s/1
  [VT] -> MATLAB Function1/1(VT)
  [PT] -> MATLAB Function1/3(PT)
  [QT] -> MATLAB Function1/2(QT)
  MATLAB Function1/1(u) -> Transfer Fcn6/1
  Transfer Fcn6/1 -> Manual Switch1/2
  Constant5/1 -> Manual Switch1/1
  Manual Switch1/1 -> Product5/2
  VUIMAX/VUIMIN/1 -> Sum5/2
  Transfer Fcn7/1 -> Sum5/1
  Constant6/1 -> Transfer Fcn7/1
  Sum5/1 -> Transfer Fcn8/1
  Transfer Fcn8/1 -> "VUELmax2/VUELmin2 "/1
  "VUELmax2/VUELmin2 "/1 -> Transfer Fcn9/1
  Transfer Fcn9/1 -> VUELmax1/VUELmin1/1
  VUELmax1/VUELmin1/1 -> Scope2/1, [VUEL]
  Constant7/1 -> Math Function2/1
  Constant8/1 -> Math Function2/2
  Math Function2/1 -> Sum6/1
  Math Function3/1 -> Sum6/2
  Constant9/1 -> Math Function3/2
  [Ifd] -> Transfer Fcn11/1
  Sum6/1 -> Gain1/1
  Gain1/1 -> SW1/2, Transfer Fcn10/1
  Transfer Fcn11/1 -> Math Function3/1
  Transfer Fcn10/1 -> Saturation/1
  Saturation/1 -> Sum7/2
  Gain2/1 -> Sum7/1
  SW1/1 -> Gain2/1
  Constant10/1 -> SW1/1
  Sum7/1 -> Saturation1/1
  Saturation1/1 -> Scope1/1, [VOEL]
  [IQ] -> Transfer Fcn12/1
  Transfer Fcn12/1 -> Sum9/2, Sum8/1
  Constant11/1 -> Sum8/2, Sum9/1
  Sum9/1 -> Gain3/1
  Gain3/1 -> Min/2
  Min/1 -> Manual Switch2/2
  MATLAB Function2/2(IUEX2) -> Manual Switch2/1
  Manual Switch2/1 -> KPUEX+KIUES/S/1
  KPUEX+KIUES/S/1 -> VSCLMAX/VSCLMIN/1
  VSCLMAX/VSCLMIN/1 -> Saturation2/1
  Saturation2/1 -> Sum10/2
  Saturation3/1 -> Sum10/1
  KPOEX+KIOEX/S1/1 -> VSCLMAX/VSCLMIN1/1
  VSCLMAX/VSCLMIN1/1 -> Saturation3/1
  Manual Switch3/1 -> KPOEX+KIOEX/S1/1
  MATLAB Function2/1(IOEX2) -> Manual Switch3/2
  Min1/1 -> Manual Switch3/1
  Sum11/1 -> Min/1, Min1/2, Scope4/1, MATLAB Function2/1(ISCLERR)
  Sum8/1 -> Gain4/1
  Gain4/1 -> Min1/1
  [IT] -> Transfer Fcn14/1, Transfer Fcn13/1
  Transfer Fcn13/1 -> Math Function4/1
  Constant12/1 -> Math Function4/2
  Math Function4/1 -> Sum11/1
  Constant13/1 -> Sum12/1, Sum11/2
  Transfer Fcn14/1 -> Sum12/2
  Sum12/1 -> Scope4/2, MATLAB Function2/2(ISCLINV)
  Sum10/1 -> Scope3/1, [VSCL]
  [VUEL] -> Max/2
  Max/1 -> Sum13/1
  [VOEL] -> Sum13/2
  Sum13/1 -> KPA+KIA/s/1
  It/1 -> [IT]
  Ifd/1 -> [IFD]
  QT/1 -> [QT]
  [QT] -> Divide/1
  [VT] -> Divide/2
  Divide/1 -> [IQ]
  PT/1 -> [PT]
  Saturation4/1 -> Product2/2
  KCL1/1 -> VRMIN/1

== system IEEE_39bus_genout/SM_master/G10/G10/Generator Measurements  ==
  note: Field Current
  note: Rotor Speed
  note: Stator Voltage
  note: Selected
      | Synchronous Machine
      | Measurement Outputs
      | (Recombined)
  note: Note:
      | This block splits the combined measurement signal into the individual parameter signals.
  note: Active Power
  note: Reactive Power
  note: Stator Current
  note: (PT2nd)
  note: (QT2nd)
  note: (It2nd)
  m : Inport
  Bus Creator : BusCreator  Inputs=7
  Bus Selector : BusSelector  OutputSignals="Mechanical.Electrical power  Pe (pu),Mechanical.Rotor speed  wm  (pu),Output active power   Peo (pu),Output reactive power  Qeo (pu),dq0 components.Stator current  id (pu),dq0 components.Stator current  iq (pu)"
  Bus Selector1 : BusSelector  OutputSignals="dq0 components.Stator voltage  vq (pu),dq0 components.Stator voltage  vd (pu)"
  Bus Selector2 : BusSelector  OutputSignals="Mechanical.Rotor speed  wm  (pu),dq0 components.Field current  ifd (pu)"
  Fcn1 : Fcn  Expr=sqrt(u(1)^2 + u(2)^2)
  Hypot : Math  Operator=hypot  SaturateOnIntegerOverflow=on
  Mux : Mux  Inputs=2
  to W : Gain  Gain=Pn
  to W1 : Gain  Gain=Pn
  to W2 : Gain  Gain=Pn
  sm : Outport  VectorParamsAs1DForOutWhenUnconnected=off
  wm : Outport  Port=2  VectorParamsAs1DForOutWhenUnconnected=off
  Vt : Outport  Port=3  VectorParamsAs1DForOutWhenUnconnected=off
  Ifd : Outport  Port=4  VectorParamsAs1DForOutWhenUnconnected=off
  It : Outport  Port=5  VectorParamsAs1DForOutWhenUnconnected=off
  PT : Outport  Port=6  VectorParamsAs1DForOutWhenUnconnected=off
  QT : Outport  Port=7  VectorParamsAs1DForOutWhenUnconnected=off
  wires:
  Fcn1/1 -> Vt/1  "Stator Voltage (pu)"
  m/1 -> Bus Selector2/1, Bus Selector1/1, Bus Selector/1
  Bus Selector2/1 -> wm/1  "<Rotor speed  wm  (pu)>"
  Bus Selector2/2 -> Ifd/1  "<Field current  ifd (pu)>"
  Hypot/1 -> It/1
  Bus Selector/6 -> Hypot/2  "<Stator current  iq (pu)>"
  Bus Selector/5 -> Hypot/1  "<Stator current  id (pu)>"
  to W2/1 -> Bus Creator/7  "Reactive Power (W)"
  to W1/1 -> Bus Creator/6  "Active Power (W)"
  Bus Selector/2 -> Bus Creator/3  "<Rotor speed  wm  (pu)>"
  Bus Creator/1 -> sm/1
  to W/1 -> Bus Creator/1  "Electrical Power (W)"
  Bus Selector/3 -> Bus Creator/4, PT/1, to W1/1  "<Output active power   Peo (pu)>"
  Bus Selector/1 -> to W/1, Bus Creator/2  "<Electrical power  Pe (pu)>"
  Bus Selector/4 -> Bus Creator/5, QT/1, to W2/1  "<Output reactive power  Qeo (pu)>"
  Bus Selector1/1 -> Mux/1  "<Stator voltage  vq (pu)>"
  Bus Selector1/2 -> Mux/2  "<Stator voltage  vd (pu)>"
  Mux/1 -> Fcn1/1

== system IEEE_39bus_genout/SM_master/G10/G10/Governor model  ==
  note: Tg = Governor time constant
  wref (pu)1 : Inport
  w (pu) : Inport  Port=2
  Input : Inport  Port=3
  1/(1+sTg) : TransferFcn  Denominator=[0.02 1]
  1/R : Gain  Gain=1/0.05
  Scope{2..6,8} (6 alike) : Scope
  Sum : Sum  Inputs=|-+
  Sum1 : Sum  Inputs=|-+
  Pmec (pu) : Outport  InitialOutput=0  VectorParamsAs1DForOutWhenUnconnected=off
  wires:
  Input/1 -> Scope6/1, Sum1/2
  1/(1+sTg)/1 -> Pmec (pu)/1, Scope5/1
  wref (pu)1/1 -> Sum/1
  Sum/1 -> 1/R/1, Scope3/1
  Sum1/1 -> 1/(1+sTg)/1, Scope2/1
  1/R/1 -> Sum1/1, Scope4/1
  w (pu)/1 -> Sum/2, Scope8/1
